simulink model "demodulationAM"  (R2019a)
settings: Solver=VariableStepAuto  StartTime=0.0  StopTime=0.9  RelTol=1e-3
libraries: dsparch4 x1
settings Model: Creator=JORGE  LastModifiedBy=JORGE

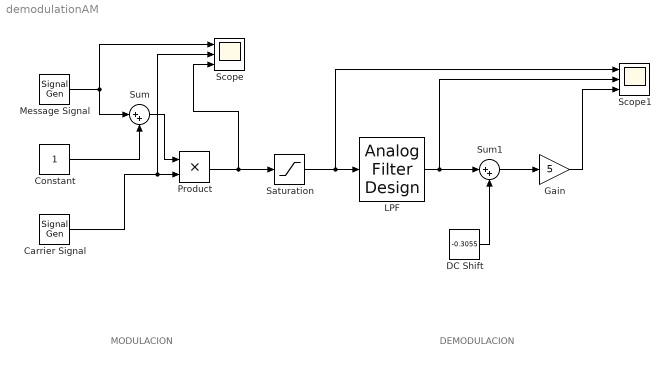
== system demodulationAM ==
  note: MODULACION
  note: DEMODULACION
  "Carrier Signal " : SignalGenerator  Frequency=100
  Constant : Constant
  DC Shift : Constant  Value=-0.3055  SampleTime=0.001
  "Gain " : Gain  Gain=5
  LPF : dsparch4/Analog Filter Design  method=Butterworth  filttype=Lowpass  N=3  Wlo=100  Whi=80  Rp=2  Rs=40
  "Message Signal " : SignalGenerator  Amplitude=0.5  Frequency=5
  Product : Product
  Saturation : Saturate  UpperLimit=3  LowerLimit=0
  Scope : Scope  NumInputPorts=3
  "Scope1 " : Scope  NumInputPorts=3
  Sum : Sum  Inputs=|++
  Sum1 : Sum  Inputs=|++
  wires:
  Saturation/1 -> "Scope1 "/1, LPF/1
  "Message Signal "/1 -> Scope/1, Sum/1
  Constant/1 -> Sum/2
  "Carrier Signal "/1 -> Scope/2, Product/2
  Sum/1 -> Product/1
  Product/1 -> Scope/3, Saturation/1
  LPF/1 -> "Scope1 "/2, Sum1/1
  "Gain "/1 -> "Scope1 "/3
  Sum1/1 -> "Gain "/1
  DC Shift/1 -> Sum1/2
